simulink subsystem "Simulation_FreeFall"  (R2024b)
settings: Solver=VariableStepAuto  StartTime=0.0  StopTime=10.0  RelTol=1e-3
model mask{poseInit=[0 0 0], vInit=[0 0 0], Ts=0.05, speedLimits=[-2 8]}
  mask prompts: poseInit "Initial position (m)"; vInit "Initial speed (m/s)"; Ts "Sampling Time (s)"; speedLimits "Speed Limits"
undefined symbols (not defined in the file): DiscIntNeverNeededParam
settings Model: Creator=marti  LastModifiedBy=marti

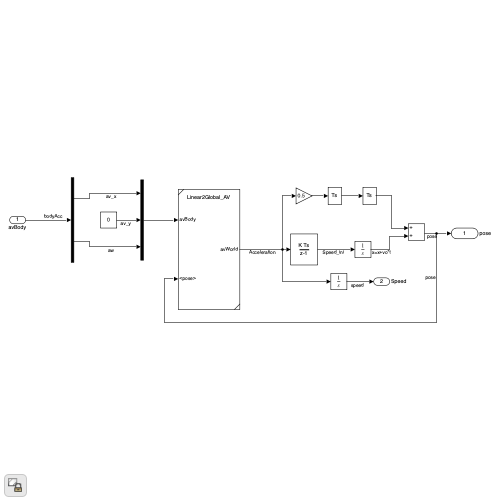
[thumbnail: Simulink's stored preview of the top-level diagram]
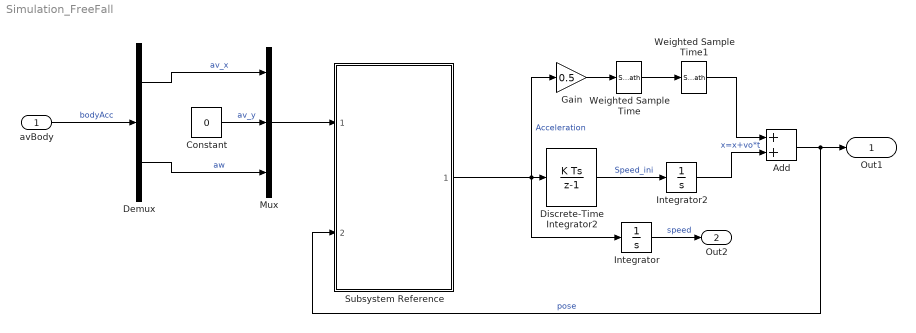
== system Simulation_FreeFall ==
  avBody : Inport  Unit=m/s^2  SampleTime=Ts
  Add : Sum
  Constant : Constant  Value=0  SampleTime=Ts
  Demux : Demux  Outputs=2
  Discrete-Time Integrator2 : DiscreteIntegrator  InitialCondition=vInit  SampleTime=Ts  ICPrevOutput=DiscIntNeverNeededParam  ICPrevScaledInput=DiscIntNeverNeededParam
  Gain : Gain  Gain=0.5
  Integrator : Integrator  InitialCondition=vInit
  Integrator2 : Integrator  InitialCondition=poseInit
  Mux : Mux  Inputs=3
  Subsystem Reference : Subsystem  ReferencedSubsystem=Linear2Global_AV
  Weighted Sample Time : SampleTimeMath  TsampMathOp=Ts Only  weightValue=1
  Weighted Sample Time1 : SampleTimeMath  TsampMathOp=Ts Only  weightValue=1
  Out1 : Outport  SignalName=pose  Unit=m  SampleTime=Ts
  Out2 : Outport  Port=2  SignalName=Speed  Unit=m/s  SampleTime=Ts
  wires:
  avBody/1 -> Demux/1  "bodyAcc"
  Subsystem Reference/1 -> Integrator/1, Gain/1, Discrete-Time Integrator2/1  "Acceleration"
  Discrete-Time Integrator2/1 -> Integrator2/1  "Speed_ini"
  Weighted Sample Time/1 -> Weighted Sample Time1/1
  Gain/1 -> Weighted Sample Time/1
  Weighted Sample Time1/1 -> Add/1
  Integrator2/1 -> Add/2  "x=x+vo*t"
  Add/1 -> Subsystem Reference/2, Out1/1  "pose"
  Integrator/1 -> Out2/1  "speed"
  Mux/1 -> Subsystem Reference/1
  Constant/1 -> Mux/2  "av_y"
  Demux/1 -> Mux/1  "av_x"
  Demux/2 -> Mux/3  "aw"
